simulink model "state_space_simulink_openloop_control101"  (R2023b)
settings: Solver=VariableStepAuto  StartTime=0.0  StopTime=endtime  RelTol=1e-3
undefined symbols (not defined in the file or in its folder): A, B, C, Cx, D, Dx
settings Model: Creator=Anthony  LastModifiedBy=Anthony Rossiter
settings DataIOCC: SaveFormat=Array
settings ModelReferenceCC: EnableRefExpFcnMdlSchedulingChecks=on

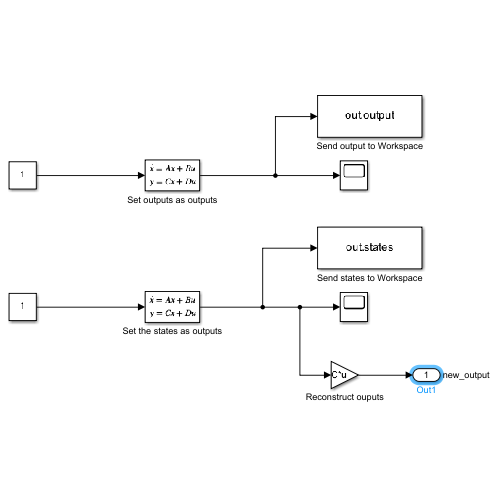
[thumbnail: Simulink's stored preview of the top-level diagram]
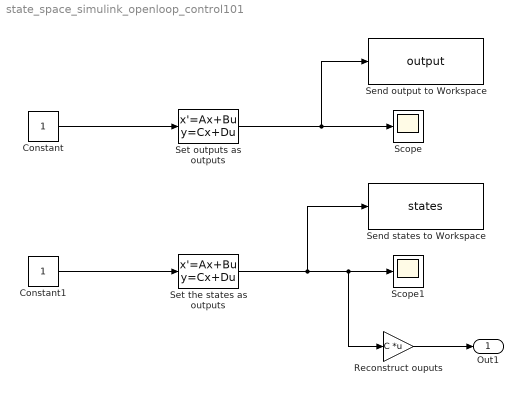
== system state_space_simulink_openloop_control101 ==
  Constant : Constant
  Constant1 : Constant
  Reconstruct ouputs : Gain  Gain=C  Multiplication=Matrix(K*u)
  Scope : Scope
  Scope1 : Scope
  Send output to Workspace : ToWorkspace  VariableName=output  SaveFormat=Structure  SampleTime=-1
  Send states to Workspace : ToWorkspace  VariableName=states  SaveFormat=Structure  SampleTime=-1
  Set outputs as outputs : StateSpace  A=A  B=B  C=C  D=D  InitialCondition=0
  Set the states as outputs : StateSpace  A=A  B=B  C=Cx  D=Dx  InitialCondition=0
  Out1 : Outport  SignalName=new_output
  wires:
  Constant/1 -> Set outputs as outputs/1
  Set outputs as outputs/1 -> Send output to Workspace/1, Scope/1
  Set the states as outputs/1 -> Reconstruct ouputs/1, Scope1/1, Send states to Workspace/1
  Constant1/1 -> Set the states as outputs/1
  Reconstruct ouputs/1 -> Out1/1
